simulink model "HoppingLEG"  (Simulink 7.7)
settings: Solver=ode3  StartTime=0.0  StopTime=inf  FixedStep=0.001  RelTol=1e-3
settings Model: Creator=Alan Mutka  LastModifiedBy=Alan Mutka

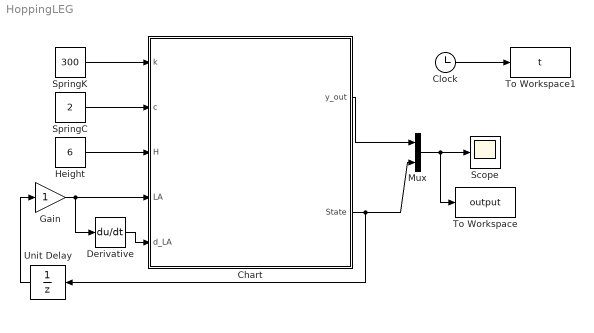
== system HoppingLEG ==
  Chart : Stateflow chart  TreatAsAtomicUnit=on
  Clock : Clock
      settings: Decimation=10
  Derivative : Derivative
  Gain : Gain
  Height : Constant  Value=6
  Mux : Mux  Inputs=3
  Scope : Scope
      settings: TimeRange=5  YMin=0  YMax=8
  SpringC : Constant  Value=2
  SpringK : Constant  Value=300
  To Workspace : ToWorkspace  VariableName=output  SampleTime=0.001  SaveFormat=Array
  To Workspace1 : ToWorkspace  VariableName=t  SampleTime=0.001  SaveFormat=Array
  Unit Delay : UnitDelay  SampleTime=-1
  wires:
  Chart/1(y_out) -> Mux/1
  Mux/1 -> Scope/1, To Workspace/1
  Derivative/1 -> Chart/5(d_LA)
  Clock/1 -> To Workspace1/1
  SpringC/1 -> Chart/2(c)
  SpringK/1 -> Chart/1(k)
  Height/1 -> Chart/3(H)
  Chart/2(State) -> Mux/3, Unit Delay/1
  Unit Delay/1 -> Gain/1
  Gain/1 -> Chart/4(LA), Derivative/1

== stateflow chart Chart ==
  settings: updateMethod=CONTINUOUS
  state Swing
    du:
    y_dot=yv;
    yv_dot=-9.81;
    //output
    y_out = y;
    State=0;
  state Stancedown
    du:
    l_dot = lv;
    lv_dot =k/mass*(l0+LA-l)-9.81-c/mass*lv+c/mass*d_LA;
    y_out = l;
    State = 1;
  (default) -> Swing : {
      | y=H;yv=0;
      | }
  Swing -> Stancedown : [y<=l0 && yv<0]
      | {
      |    //ako pada prebaci
      |     l = y;
      |     lv = yv;
      |
      | }
  Stancedown -> Swing : [l>l0 && lv>0]
      | {
      |    //ako pada prebaci
      | y=l;
      | yv = lv;
      |
      | }
  data: l local double; yv local double; y_out output double; y local double; lv local double; k input double =800; mass constant double =1; l0 constant double =3; c input double =6; H input double; LA input double =0; d_LA input double =0; State output double
  data l settings: updateMethod=SF_CONTINUOUS_TIME_DATA
  data yv settings: updateMethod=SF_CONTINUOUS_TIME_DATA
  data y settings: updateMethod=SF_CONTINUOUS_TIME_DATA
  data lv settings: updateMethod=SF_CONTINUOUS_TIME_DATA
  data H settings: updateMethod=SF_CONTINUOUS_TIME_DATA
